simulink model "blockdemo"  (Simulink 6.3)
settings: Solver=FixedStepDiscrete  StartTime=0  StopTime=30  MaxStep=1  RelTol=1e-3
InitFcn:
  | %% DSPBuilder Start
  | alt_dspbuilder_update_model(bdroot)
  | %% DSPBuilder End
libraries: allblocks_alteradspbuilder2 x8
settings Model: Creator=mjervis  LastModifiedBy=delphick
settings OptimizationCC: BooleanDataType=off  InlineInvariantSignals=on
settings DebuggingCC: SolverPrmCheckMsg=none
settings HardwareCC: TargetUnknown=on

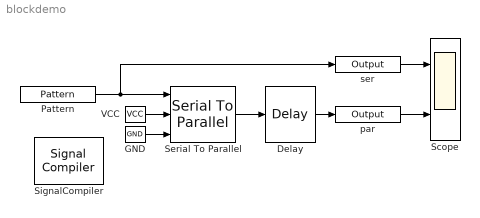
== system blockdemo ==
  Delay : allblocks_alteradspbuilder2/Delay  pipeline=1  ClockPhase=1000  use_ena=off  use_sclr=off
      settings: AttributesFormatString=ClockPhase = %<ClockPhase>\nPipeline = %<pipeline>
  GND : allblocks_alteradspbuilder2/GND  SpecifyClock=off
  Pattern : allblocks_alteradspbuilder2/Pattern  Sequence=100111010  SpecifyClock=off  use_ena=off  use_sclr=off
  Scope : Scope  NumInputPorts=2
      settings: TimeRange=30  YMin=-0.5~0  YMax=1.5~8
  Serial To Parallel : allblocks_alteradspbuilder2/Serial To Parallel  BusType=Unsigned Integer  bwl=3  bwr=0  msbfirsttext=LSB First  msbfirst=0
      settings: AttributesFormatString=%<msbfirsttext>\n%<BusType>
  SignalCompiler : allblocks_alteradspbuilder2/Signal Compiler  DeviceFamily=Cyclone IV GX  DeviceName=AUTO  EnableSignalTap=off  SignalTapDepth=128  UseBoardBlock=off  StpUseDefaultClock=on  StpClock=clock
  VCC : allblocks_alteradspbuilder2/VCC  SpecifyClock=off
  par : allblocks_alteradspbuilder2/Output  iofile=C:\workspace_clean\Documentation\DesignExamples\Tutorials\UnitBlocks\Storage\SerialToParallel\tb_blockdemo\blockdemo_par.capture  BusType=Inferred  bwl=4  bwr=0  PORTTYPE=Output
  ser : allblocks_alteradspbuilder2/Output  iofile=C:\workspace_clean\Documentation\DesignExamples\Tutorials\UnitBlocks\Storage\SerialToParallel\tb_blockdemo\blockdemo_ser.capture  BusType=Single Bit  bwl=1  bwr=0  PORTTYPE=Output
  wires:
  Pattern/1 -> Serial To Parallel/1, ser/1
  VCC/1 -> Serial To Parallel/2
  GND/1 -> Serial To Parallel/3
  Serial To Parallel/1 -> Delay/1
  ser/1 -> Scope/1
  par/1 -> Scope/2
  Delay/1 -> par/1
